simulink model "BBrakeError"  (R2024b)
settings: configuration reference "STM32H7_Config" (kept outside this file)
undefined symbols (not defined in the file): pBrakeErrorHigh, pBrakeErrorLow, pBrakeOverlapThreshold, tSystemsTask
libraries: simulink x3
settings Model: DataDictionary=Master_Dictionary.sldd  EnableAccessToBaseWorkspace=off  Creator=torni  LastModifiedBy=William
settings ConfigSetRef: SourceName=STM32H7_Config

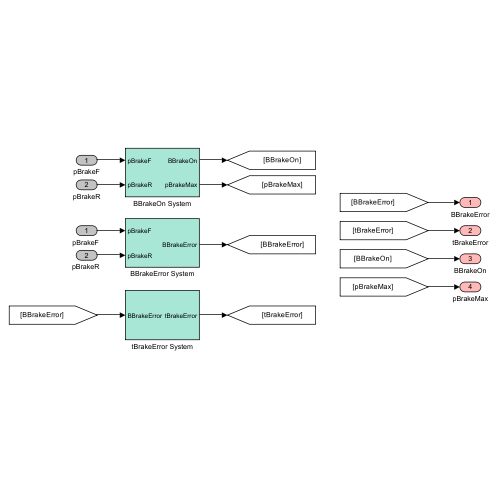
[thumbnail: Simulink's stored preview of the top-level diagram]
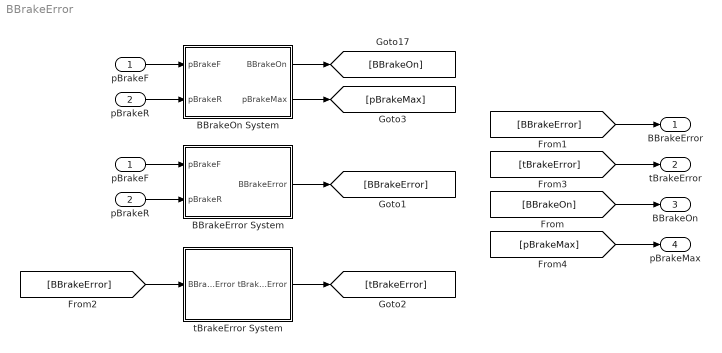
== system BBrakeError ==
  pBrakeF : Inport  OutDataTypeStr=double
  pBrakeR : Inport  Port=2  OutDataTypeStr=double
  BBrakeError System : Subsystem
  BBrakeOn System : Subsystem
  "pBrakeF " : InportShadow  OutDataTypeStr=double
  "pBrakeR " : InportShadow  Port=2  OutDataTypeStr=double
  tBrakeError System : Subsystem
  BBrakeError : Outport  OutDataTypeStr=boolean  VectorParamsAs1DForOutWhenUnconnected=off
  tBrakeError : Outport  Port=2  OutDataTypeStr=double  VectorParamsAs1DForOutWhenUnconnected=off
  BBrakeOn : Outport  Port=3  OutDataTypeStr=boolean  VectorParamsAs1DForOutWhenUnconnected=off
  pBrakeMax : Outport  Port=4  OutDataTypeStr=double  VectorParamsAs1DForOutWhenUnconnected=off
  wires:
  pBrakeF/1 -> BBrakeOn System/1(pBrakeF)
  pBrakeR/1 -> BBrakeOn System/2(pBrakeR)
  "pBrakeF "/1 -> BBrakeError System/1(pBrakeF)
  "pBrakeR "/1 -> BBrakeError System/2(pBrakeR)
  BBrakeOn System/1(BBrakeOn) -> [BBrakeOn]
  [BBrakeOn] -> BBrakeOn/1
  BBrakeError System/1(BBrakeError) -> [BBrakeError]
  [BBrakeError] -> BBrakeError/1
  [BBrakeError] -> tBrakeError System/1(BBrakeError)
  tBrakeError System/1(tBrakeError) -> [tBrakeError]
  [tBrakeError] -> tBrakeError/1
  BBrakeOn System/2(pBrakeMax) -> [pBrakeMax]
  [pBrakeMax] -> pBrakeMax/1

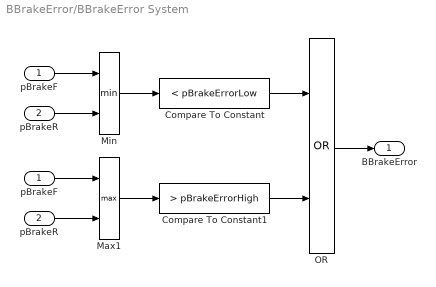
== system BBrakeError/BBrakeError System ==
  pBrakeF : Inport  OutDataTypeStr=double
  pBrakeR : Inport  Port=2  OutDataTypeStr=double
  Compare To Constant : simulink/Logic and Bit Operations/Compare To Constant  relop=<  const=pBrakeErrorLow  OutDataTypeStr=boolean
  Compare To Constant1 : simulink/Logic and Bit Operations/Compare To Constant  relop=>  const=pBrakeErrorHigh  OutDataTypeStr=boolean
  Max1 : MinMax  Function=max  Inputs=2
  Min : MinMax  Inputs=2
  OR : Logic  Operator=OR  AllPortsSameDT=off  OutDataTypeStr=boolean
  "pBrakeF " : InportShadow  OutDataTypeStr=double
  "pBrakeR " : InportShadow  Port=2  OutDataTypeStr=double
  BBrakeError : Outport  OutDataTypeStr=boolean  VectorParamsAs1DForOutWhenUnconnected=off
  wires:
  Compare To Constant/1 -> OR/1
  OR/1 -> BBrakeError/1
  pBrakeF/1 -> Min/1
  Max1/1 -> Compare To Constant1/1
  Min/1 -> Compare To Constant/1
  "pBrakeR "/1 -> Max1/2
  "pBrakeF "/1 -> Max1/1
  Compare To Constant1/1 -> OR/2
  pBrakeR/1 -> Min/2

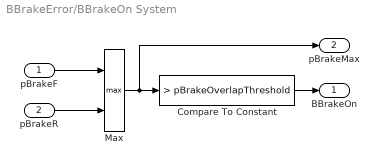
== system BBrakeError/BBrakeOn System ==
  pBrakeF : Inport  OutDataTypeStr=double
  pBrakeR : Inport  Port=2  OutDataTypeStr=double
  Compare To Constant : simulink/Logic and Bit Operations/Compare To Constant  relop=>  const=pBrakeOverlapThreshold  OutDataTypeStr=boolean
  Max : MinMax  Function=max  Inputs=2
  BBrakeOn : Outport  OutDataTypeStr=boolean  VectorParamsAs1DForOutWhenUnconnected=off
  pBrakeMax : Outport  Port=2  OutDataTypeStr=double  VectorParamsAs1DForOutWhenUnconnected=off
  wires:
  pBrakeR/1 -> Max/2
  Max/1 -> Compare To Constant/1, pBrakeMax/1
  Compare To Constant/1 -> BBrakeOn/1
  pBrakeF/1 -> Max/1

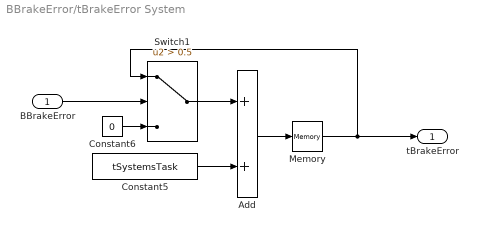
== system BBrakeError/tBrakeError System ==
  BBrakeError : Inport  OutDataTypeStr=boolean
  Add : Sum
  Constant5 : Constant  Value=tSystemsTask
  Constant6 : Constant  Value=0
  Memory : Memory  InheritSampleTime=on
  Switch1 : Switch  Criteria=u2 > Threshold  Threshold=0.5  SaturateOnIntegerOverflow=off  InputSameDT=off
  tBrakeError : Outport  OutDataTypeStr=double  VectorParamsAs1DForOutWhenUnconnected=off
  wires:
  Memory/1 -> Switch1/1, tBrakeError/1
  Constant6/1 -> Switch1/3
  Constant5/1 -> Add/2
  Add/1 -> Memory/1
  BBrakeError/1 -> Switch1/2
  Switch1/1 -> Add/1
